simulink model "CR_Circuit_high_pass_filter"  (R2022a)
settings: Solver=FixedStepAuto  StartTime=0.0  StopTime=10.0  FixedStep=0.001  RelTol=1e-3
libraries: simulink x5
settings Model: Creator=Kieran  LastModifiedBy=Kieran

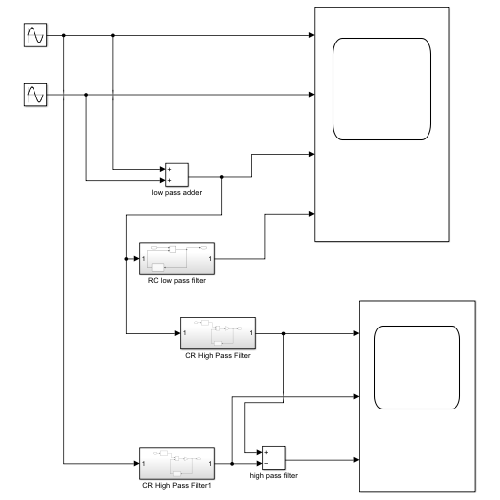
[thumbnail: Simulink's stored preview of the top-level diagram]
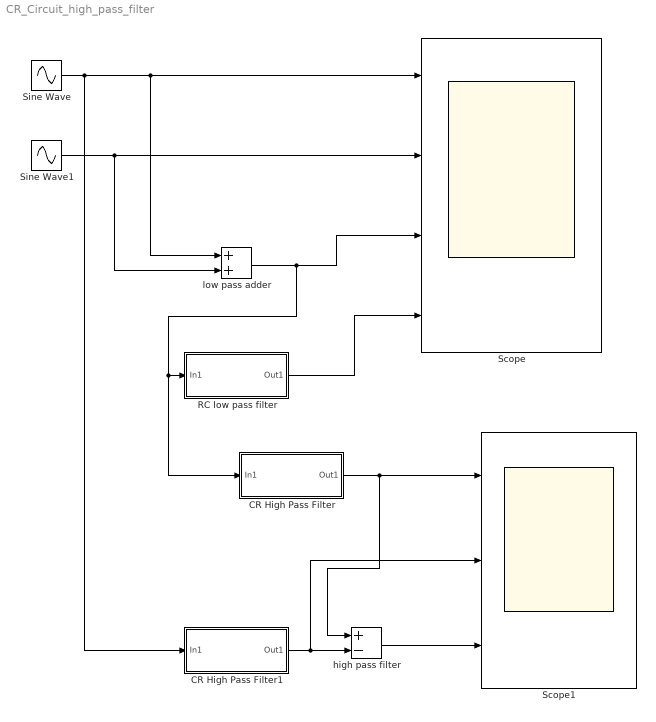
== system CR_Circuit_high_pass_filter ==
  CR High Pass Filter : Subsystem
  CR High Pass Filter1 : Subsystem
  RC low pass filter : Subsystem
  Scope : Scope  NumInputPorts=4
  Scope1 : Scope  NumInputPorts=3
  Sine Wave : Sin  Amplitude=50  SampleTime=0
  Sine Wave1 : Sin  Amplitude=5  Frequency=10  SampleTime=0
  high pass filter : Sum  Inputs=+-
  low pass adder : Sum
  wires:
  Sine Wave/1 -> CR High Pass Filter1/1(In1), low pass adder/1, Scope/1
  Sine Wave1/1 -> low pass adder/2, Scope/2
  low pass adder/1 -> CR High Pass Filter/1(In1), RC low pass filter/1(In1), Scope/3
  RC low pass filter/1(Out1) -> Scope/4
  CR High Pass Filter/1(Out1) -> high pass filter/1, Scope1/1
  high pass filter/1 -> Scope1/3
  CR High Pass Filter1/1(Out1) -> Scope1/2, high pass filter/2

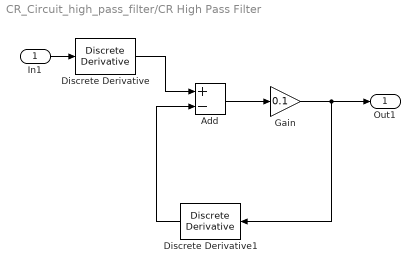
== system CR_Circuit_high_pass_filter/CR High Pass Filter ==
  In1 : Inport
  Add : Sum  Inputs=+-
  Discrete Derivative : simulink/Discrete/Discrete Derivative  gainval=1.0  ICPrevScaledInput=0.0  OutMin=[]  OutMax=[]  OutDataType=fixdt(1, 16)  OutScaling=2^-10  DoSatur=off
  Discrete Derivative1 : simulink/Discrete/Discrete Derivative  gainval=1.0  ICPrevScaledInput=0.0  OutMin=[]  OutMax=[]  OutDataType=fixdt(1, 16)  OutScaling=2^-10  DoSatur=off
  Gain : Gain  Gain=0.1
  Out1 : Outport
  wires:
  Add/1 -> Gain/1
  Gain/1 -> Discrete Derivative1/1, Out1/1
  In1/1 -> Discrete Derivative/1
  Discrete Derivative/1 -> Add/1
  Discrete Derivative1/1 -> Add/2

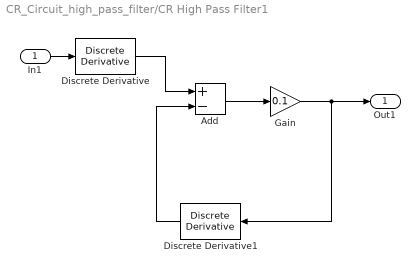
== system CR_Circuit_high_pass_filter/CR High Pass Filter1 ==
  In1 : Inport
  Add : Sum  Inputs=+-
  Discrete Derivative : simulink/Discrete/Discrete Derivative  gainval=1.0  ICPrevScaledInput=0.0  OutMin=[]  OutMax=[]  OutDataType=fixdt(1, 16)  OutScaling=2^-10  DoSatur=off
  Discrete Derivative1 : simulink/Discrete/Discrete Derivative  gainval=1.0  ICPrevScaledInput=0.0  OutMin=[]  OutMax=[]  OutDataType=fixdt(1, 16)  OutScaling=2^-10  DoSatur=off
  Gain : Gain  Gain=0.1
  Out1 : Outport
  wires:
  Add/1 -> Gain/1
  Gain/1 -> Discrete Derivative1/1, Out1/1
  In1/1 -> Discrete Derivative/1
  Discrete Derivative/1 -> Add/1
  Discrete Derivative1/1 -> Add/2

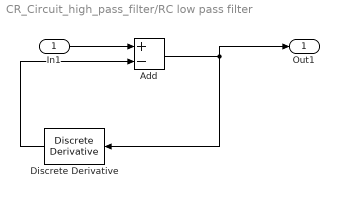
== system CR_Circuit_high_pass_filter/RC low pass filter ==
  In1 : Inport
  Add : Sum  Inputs=+-
  Discrete Derivative : simulink/Discrete/Discrete Derivative  gainval=1.0  ICPrevScaledInput=0.0  OutMin=[]  OutMax=[]  OutDataType=fixdt(1, 16)  OutScaling=2^-10  DoSatur=off
  Out1 : Outport
  wires:
  In1/1 -> Add/1
  Discrete Derivative/1 -> Add/2
  Add/1 -> Discrete Derivative/1, Out1/1
